simulink model "arduino_xcponserial_Teensy_2025b"  (R2025b)
settings: Solver=FixedStepAuto  StartTime=0.0  StopTime=Inf  RelTol=1e-3  EnableMultiTasking=on
model workspace (MAT data in the model file):
  CONST_AMPLITUDE = Simulink.Parameter
  CONST_AMPLITUDE.Value = 1
  CONST_AMPLITUDE.Complexity = 'real'
  CONST_AMPLITUDE.Dimensions = [1 1]
  CONST_AMPLITUDE.DataType = 'single'
  Counter = Simulink.Signal
  Counter.Dimensions = -1
  Counter.DimensionsMode = 'auto'
  Counter.Complexity = 'auto'
  Counter.SampleTime = -1
  Counter.SamplingMode = 'auto'
  Counter.DataType = 'uint16'
  PULSE_AMPLITUDE = Simulink.Parameter
  PULSE_AMPLITUDE.Value = 2
  PULSE_AMPLITUDE.Complexity = 'real'
  PULSE_AMPLITUDE.Dimensions = [1 1]
  PULSE_AMPLITUDE.DataType = 'single'
  Pulse = Simulink.Signal
  Pulse.Dimensions = -1
  Pulse.DimensionsMode = 'auto'
  Pulse.Complexity = 'auto'
  Pulse.SampleTime = -1
  Pulse.SamplingMode = 'auto'
  Pulse.DataType = 'uint32'
  STEP_PARAM = Simulink.Parameter
  STEP_PARAM.Value = 1
  STEP_PARAM.Complexity = 'real'
  STEP_PARAM.Dimensions = [1 1]
  STEP_PARAM.DataType = 'uint16'
  Sine_Wave = Simulink.Signal
  Sine_Wave.Dimensions = -1
  Sine_Wave.DimensionsMode = 'auto'
  Sine_Wave.Complexity = 'auto'
  Sine_Wave.SampleTime = -1
  Sine_Wave.SamplingMode = 'auto'
  Sine_Wave.DataType = 'single'
  constSig = Simulink.Signal
  constSig.Dimensions = -1
  constSig.DimensionsMode = 'auto'
  constSig.Complexity = 'auto'
  constSig.SampleTime = -1
  constSig.SamplingMode = 'auto'
  constSig.DataType = 'single'
settings Model: ExtModeTrigDuration=2  Creator=The MathWorks, Inc.  LastModifiedBy=benir
settings SolverCC: AlgebraicLoopSolver=TrustRegion  AutoInsertRateTranBlk=on  MaxZcPerStep=1.0
settings OptimizationCC: EnhancedBackFolding=on  PassReuseOutputArgsAs=Individual arguments  ZeroExternalMemoryAtStartup=off  ZeroInternalMemoryAtStartup=off  MaxStackSize=64  OptimizeBlockOrder=speed  DifferentSizesBufferReuse=on  OptimizationCustomize=off  EfficientTunableParamExpr=on
settings DebuggingCC: ParameterTunabilityLossMsg=error  UnconnectedInputMsg=warning  UnconnectedOutputMsg=warning  UnconnectedLineMsg=warning
settings HardwareCC: ProdBitPerPointer=32.0  ProdBitPerSizeT=32.0  ProdBitPerPtrDiffT=32.0  ProdLargestAtomicInteger=Long  ProdLargestAtomicFloat=Double  ProdWordSize=32.0  ProdHWDeviceType=ARM Compatible->ARM Cortex
settings ModelReferenceCC: EnableRefExpFcnMdlSchedulingChecks=on
settings SFSimCC: MATLABDynamicMemAlloc=off
settings RTWCC: SystemTargetFile=ert.tlc  HardwareBoard=Teensy 4.1 (Arduino Compatible)  TemplateMakefile=ert_default_tmf  Toolchain=Arduino ARM M7  BuildConfiguration=Faster Runs  GPUComputeCapability=3.5  DLArmComputeVersion=19.05  Description=Embedded Coder
settings CodeAppCC: ForceParamTrailComments=on  IgnoreCustomStorageClasses=off  OperatorAnnotations=on  SimulinkDataObjDesc=on  SFDataObjDesc=on  InsertBlockDesc=on
settings ERTTargetCC: ExtModeTransport=3.0  ExtModeStaticAlloc=on  ExtModeAutomaticAllocSize=off  ExtModeStaticAllocSize=65536.0  ExtModeMexFile=ext_xcp  ExtModeIntrfLevel=Level2 - Open  InlinedParameterPlacement=Hierarchical  DynamicArrayContainerType=coder::array  SupportContinuousTime=on  SupportNonInlinedSFcns=on  SupportVariableSizeSignals=on

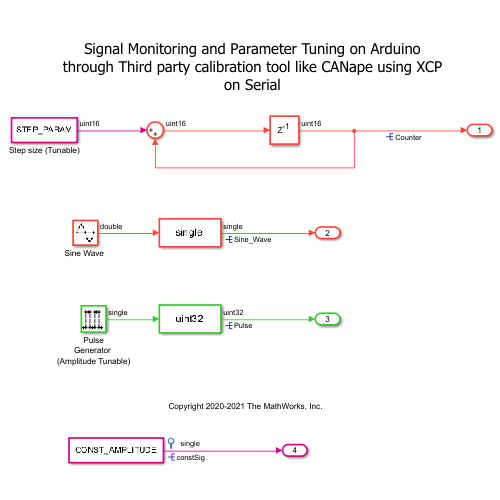
[thumbnail: Simulink's stored preview of the top-level diagram]
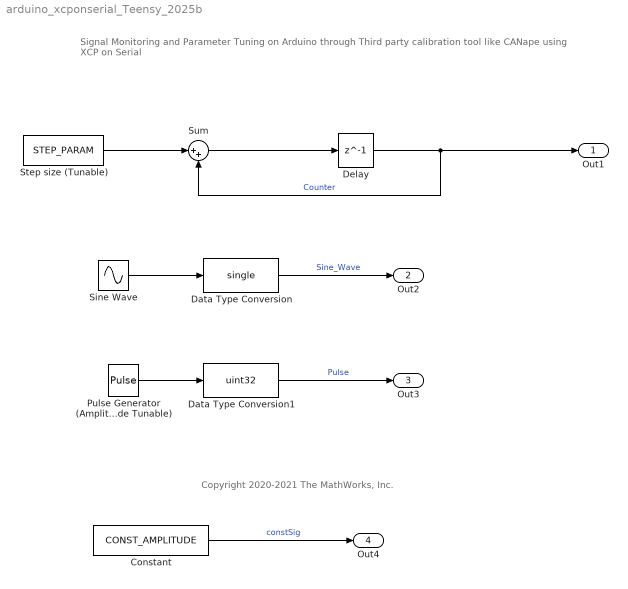
== system arduino_xcponserial_Teensy_2025b ==
  note: Copyright 2020-2021 The MathWorks, Inc.
  note: Signal Monitoring and Parameter Tuning on Arduino through Third party calibration tool like CANape using XCP on Serial
  Constant : Constant  Value=CONST_AMPLITUDE
  Data Type Conversion : DataTypeConversion  OutDataTypeStr=single  SaturateOnIntegerOverflow=off  RndMeth=Floor
  Data Type Conversion1 : DataTypeConversion  OutDataTypeStr=uint32  SaturateOnIntegerOverflow=off  RndMeth=Floor
  Delay : Delay  DelayLength=1
  Pulse Generator (Amplitude Tunable) : DiscretePulseGenerator  Amplitude=PULSE_AMPLITUDE  Period=10  PulseWidth=5  SampleTime=0.2
  "Sine Wave " : Sin  SineType=Sample based  Amplitude=5  Samples=20  SampleTime=0.1
  Step size (Tunable) : Constant  Value=STEP_PARAM
  Sum : Sum  Inputs=|++
  Out1 : Outport
  Out2 : Outport  Port=2
  Out3 : Outport  Port=3
  Out4 : Outport  Port=4
  wires:
  Step size (Tunable)/1 -> Sum/1
  Sum/1 -> Delay/1
  Delay/1 -> Sum/2, Out1/1  "Counter"
  Pulse Generator (Amplitude Tunable)/1 -> Data Type Conversion1/1
  "Sine Wave "/1 -> Data Type Conversion/1
  Data Type Conversion/1 -> Out2/1  "Sine_Wave"
  Data Type Conversion1/1 -> Out3/1  "Pulse"
  Constant/1 -> Out4/1  "constSig"
